simulink model "prj"  (R2023b)
settings: Solver=VariableStepAuto  StartTime=0.0  StopTime=100.0  RelTol=1e-3
undefined symbols (not defined in the file): A_lat, A_long, B_lat, B_long, C, Car_weight, D, Rain_rate, Road_condition, Wind_speed
libraries: slctrl_adaptive x2
settings Model: Creator=setak  LastModifiedBy=setak

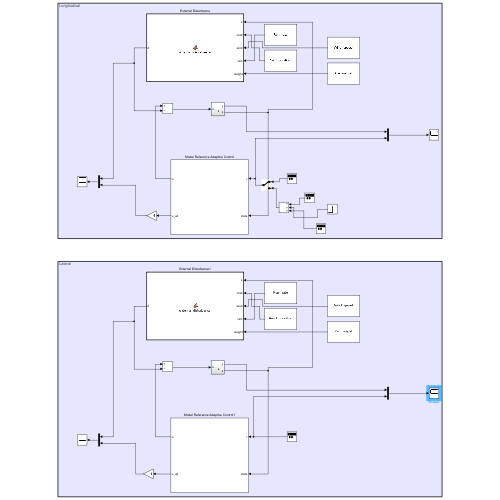
[thumbnail: Simulink's stored preview of the top-level diagram]
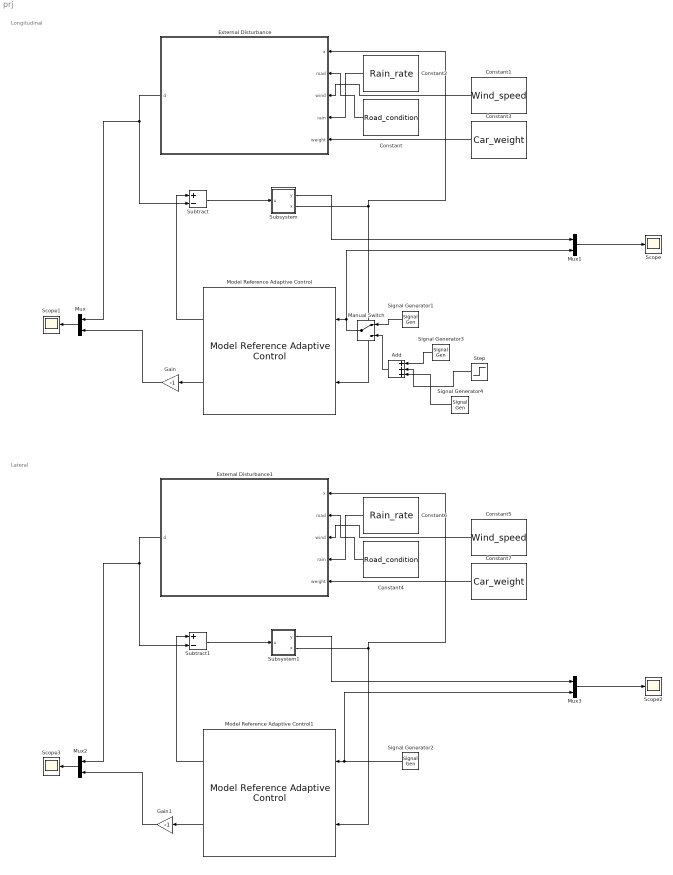
== system prj ==
  note: Longitudinal
  note: Lateral
  Add : Sum  Inputs=+++
  Constant : Constant  Value=Road_condition
  Constant1 : Constant  Value=Wind_speed
  Constant2 : Constant  Value=Rain_rate
  Constant3 : Constant  Value=Car_weight
  Constant4 : Constant  Value=Road_condition
  Constant5 : Constant  Value=Wind_speed
  Constant6 : Constant  Value=Rain_rate
  Constant7 : Constant  Value=Car_weight
  External Disturbance : MATLAB Function  TreatAsAtomicUnit=on
  External Disturbance1 : MATLAB Function  TreatAsAtomicUnit=on
  Gain : Gain  Gain=-1
  Gain1 : Gain  Gain=-1
  Manual Switch : ManualSwitch
  Model Reference Adaptive Control : slctrl_adaptive/Model Reference Adaptive Control  selectType=Direct  A=A_long  B=B_long  Ahat=0  ALrEnable=on  gamma_a=1  ALrEnableMod=on  Bhat=1  BLrEnable=on  gamma_b=1  BLrEnableMod=on  externalKtauEnable=off  k_tau=-1  estParamOutput=off  Am=Am_long  Bm=Bm_long  kx=Kx_long  FBLrEnable=on  gamma_kx=gamma_w  FBLrEnableMod=on  kr=Kr_long  FFLrEnable=on  gamma_kr=gamma_w  FFLrEnableMod=on  AdaptEnable=on  gamma=gamma_w  WLrEnableMod=on  Q=Q  FeatureTypeOptions=Radial Basis Function  shlHiddenLayerSize=10  gamma_V=0.1  nCen=30  cSpanMin=-1  cSpanMax=1  cSig=5  adaptiveCntrlOutport=on  modChoice=None  sigma_val=0.1
      settings: LibrarySourceBlock=slctrlblks/Adaptive Control/Model Reference Adaptive Control
  Model Reference Adaptive Control1 : slctrl_adaptive/Model Reference Adaptive Control  selectType=Direct  A=A_lat  B=B_lat  Ahat=0  ALrEnable=on  gamma_a=1  ALrEnableMod=on  Bhat=1  BLrEnable=on  gamma_b=1  BLrEnableMod=on  externalKtauEnable=off  k_tau=-1  estParamOutput=off  Am=Am_lat  Bm=Bm_lat  kx=Kx_lat  FBLrEnable=on  gamma_kx=gamma_w  FBLrEnableMod=on  kr=Kr_lat  FFLrEnable=on  gamma_kr=gamma_w  FFLrEnableMod=on  AdaptEnable=on  gamma=gamma_w  WLrEnableMod=on  Q=Q  FeatureTypeOptions=Radial Basis Function  shlHiddenLayerSize=10  gamma_V=0.1  nCen=30  cSpanMin=-1  cSpanMax=1  cSig=5  adaptiveCntrlOutport=on  modChoice=None  sigma_val=0.1
      settings: LibrarySourceBlock=slctrlblks/Adaptive Control/Model Reference Adaptive Control
  Mux{,1..3} (4 alike) : Mux  Inputs=2
  Scope{,1..3} (4 alike) : Scope
  Signal Generator1 : SignalGenerator  Frequency=0.5  Units=rad/sec
  Signal Generator2 : SignalGenerator  Units=rad/sec
  Signal Generator3 : SignalGenerator  Frequency=0.5  Units=rad/sec
  Signal Generator4 : SignalGenerator  Frequency=2  Units=rad/sec
  Step : Step  SampleTime=0
  Subsystem : Subsystem
  Subsystem1 : Subsystem
  Subtract : Sum  Inputs=+-
  Subtract1 : Sum  Inputs=+-
  wires:
  Constant/1 -> External Disturbance/2(road)
  Constant1/1 -> External Disturbance/3(wind)
  Constant2/1 -> External Disturbance/4(rain)
  Constant3/1 -> External Disturbance/5(weight)
  Subtract/1 -> Subsystem/1(u)
  Subsystem/2(x) -> External Disturbance/1(x), Model Reference Adaptive Control/2
  External Disturbance/1(d) -> Mux/1, Subtract/2
  Mux/1 -> Scope1/1
  Mux1/1 -> Scope/1
  Model Reference Adaptive Control/2 -> Gain/1
  Model Reference Adaptive Control/1 -> Subtract/1
  Subsystem/1(y) -> Mux1/1
  Subtract1/1 -> Subsystem1/1(u)
  Subsystem1/2(x) -> External Disturbance1/1(x), Model Reference Adaptive Control1/2
  Model Reference Adaptive Control1/2 -> Gain1/1
  Constant5/1 -> External Disturbance1/3(wind)
  Model Reference Adaptive Control1/1 -> Subtract1/1
  Signal Generator2/1 -> Mux3/2, Model Reference Adaptive Control1/1
  Subsystem1/1(y) -> Mux3/1
  Constant6/1 -> External Disturbance1/4(rain)
  Constant4/1 -> External Disturbance1/2(road)
  Mux2/1 -> Scope3/1
  Mux3/1 -> Scope2/1
  Constant7/1 -> External Disturbance1/5(weight)
  External Disturbance1/1(d) -> Mux2/1, Subtract1/2
  Gain/1 -> Mux/2
  Gain1/1 -> Mux2/2
  Signal Generator3/1 -> Add/1
  Step/1 -> Add/2
  Signal Generator4/1 -> Add/3
  Signal Generator1/1 -> Manual Switch/1
  Add/1 -> Manual Switch/2
  Manual Switch/1 -> Mux1/2, Model Reference Adaptive Control/1

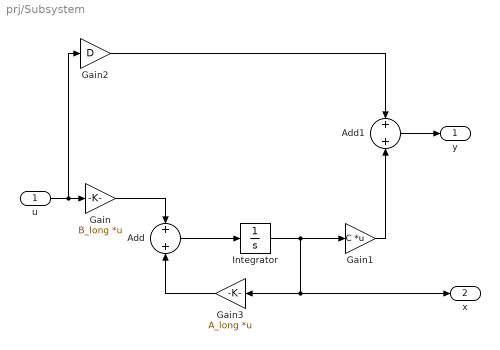
== system prj/Subsystem ==
  u : Inport
  Add : Sum  Inputs=+|+
  Add1 : Sum  Inputs=+|+
  Gain : Gain  Gain=B_long  Multiplication=Matrix(K*u)
  Gain1 : Gain  Gain=C  Multiplication=Matrix(K*u)
  Gain2 : Gain  Gain=D
  Gain3 : Gain  Gain=A_long  Multiplication=Matrix(K*u)
  Integrator : Integrator
  y : Outport
  x : Outport  Port=2
  wires:
  Add/1 -> Integrator/1
  Gain1/1 -> Add1/2
  Gain3/1 -> Add/2
  u/1 -> Gain2/1, Gain/1
  Integrator/1 -> x/1, Gain3/1, Gain1/1
  Gain/1 -> Add/1
  Add1/1 -> y/1
  Gain2/1 -> Add1/1

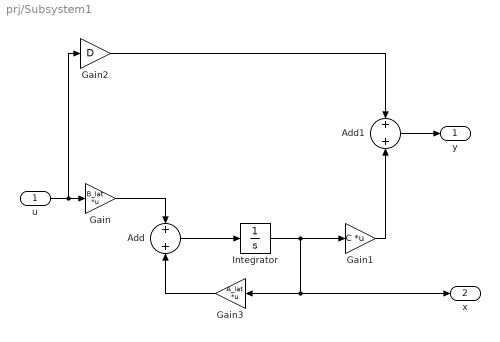
== system prj/Subsystem1 ==
  u : Inport
  Add : Sum  Inputs=+|+
  Add1 : Sum  Inputs=+|+
  Gain : Gain  Gain=B_lat  Multiplication=Matrix(K*u)
  Gain1 : Gain  Gain=C  Multiplication=Matrix(K*u)
  Gain2 : Gain  Gain=D
  Gain3 : Gain  Gain=A_lat  Multiplication=Matrix(K*u)
  Integrator : Integrator
  y : Outport
  x : Outport  Port=2
  wires:
  Add/1 -> Integrator/1
  Gain1/1 -> Add1/2
  Gain3/1 -> Add/2
  u/1 -> Gain2/1, Gain/1
  Integrator/1 -> x/1, Gain3/1, Gain1/1
  Gain/1 -> Add/1
  Add1/1 -> y/1
  Gain2/1 -> Add1/1

== matlab function prj/External Disturbance1 ==
  data: x input size=2; road input; wind input; d output size=1; rain input; weight input
function d = external_disturbance(x, road, wind, rain, weight)
% x: scalar longitudinal speed
% road, wind, rain, weight: scalar environment inputs

% Environmental weights (tunable)
alpha = 0.05;  % road condition impact
beta  = 2;  % wind effect
gamma = 30;  % rain effect
delta = 20; % car weight effect

v = x(1);  % speed

% Disturbance based on environment and speed
d_long = ...
    alpha * (100 - road) * abs(v) + ...
    beta  * wind * sign(v) + ...
    gamma * rain * abs(v) + ...
    delta * weight * 9.81 / 1000;

% Output disturbance vector (for 2nd order system)
d = d_long;

== matlab function prj/External Disturbance ==
  data: x input size=2; road input; wind input; d output size=1; rain input; weight input
function d = external_disturbance(x, road, wind, rain, weight)
% x: scalar longitudinal speed
% road, wind, rain, weight: scalar environment inputs

% Environmental weights (tunable)
alpha = 0.5;  % road condition impact
beta  = 15;  % wind effect
gamma = 3;  % rain effect
delta = 20; % car weight effect

v = x(1);  % speed

% Disturbance based on environment and speed
d_long = ...
    alpha * (100 - road) * abs(v) + ...
    beta  * wind * sign(v) + ...
    gamma * rain * abs(v) + ...
    delta * weight * 9.81 / 1000;

% Output disturbance vector (for 2nd order system)
d = d_long;
